simulink model "e11_cascade"  (R2020a)
settings: Solver=FixedStepAuto  StartTime=0.0  StopTime=options.T_train  RelTol=1e-3  AbsTol=1e-6
model workspace (MATLAB code in the model file):
  | scd_aero_guid_dat
undefined symbols (not defined in the file or in its folder): Cm_alpha, Cm_el, Cm_q, Cx_alpha, Cz_alpha, Cz_el, d_ref, DiscIntNeverNeededParam, g, h_ini, options, S_ref, Thrust, x_ini
libraries: neural x86, aerospace x6, simulink x1
(part 1 of 5)
settings Model: ExtModeTrigMode=oneshot  ExtModeArmWhenConnect=off  ExtModeAutoUpdateStatusClock=off  Creator=The MathWorks, Inc.  LastModifiedBy=kekatos
settings SolverCC: AutoScaleAbsTol=off
settings DataIOCC: SaveFormat=Array  SaveOutput=off  SignalLogging=off  SaveTime=off  ReturnWorkspaceOutputs=off  SignalLoggingName=sigsOut
settings OptimizationCC: BlockReduction=off  BooleanDataType=off  DefaultParameterBehavior=Inlined  InlineInvariantSignals=on  BufferReuse=off  ExpressionDepthLimit=2147483647  InitFltsAndDblsToZero=on  LifeSpan=inf
settings DebuggingCC: SaveWithParameterizedLinksMsg=none  UnderspecifiedInitializationDetection=Classic  MergeDetectMultiDrivingBlocksExec=none  CheckExecutionContextPreStartOutputMsg=on  CheckExecutionContextRuntimeOutputMsg=on  SignalResolutionControl=TryResolveAllWithWarning  MultiTaskDSMMsg=warning  FcnCallInpInsideContextMsg=warning  StateNameClashWarn=warning  SFUnexpectedBacktrackingDiag=warning  SFNoUnconditionalDefaultTransitionDiag=warning  SFExecutionAtInitializationDiag=none  ArithmeticOperatorsInVariantConditions=warning
settings HardwareCC: ProdBitPerPointer=32  ProdBitPerSizeT=32  ProdBitPerPtrDiffT=32  ProdLargestAtomicFloat=None  ProdIntDivRoundTo=Undefined  ProdEndianess=Unspecified  ProdWordSize=32  ProdHWDeviceType=32-bit Generic  TargetUnknown=on
settings ModelReferenceCC: UpdateModelReferenceTargets=IfOutOfDate  PropagateSignalLabelsOutOfModel=off
settings SFSimCC: SimUseLocalCustomCode=off  CustomCodeUndefinedFunction=UseInterfaceOnly
settings RTWCC: RTWUseLocalCustomCode=off
settings CodeAppCC: StateflowObjectComments=on
settings GRTTargetCC: TargetFcnLib=ansi_tfl_tmw.mat  TargetLangStandard=C89/C90 (ANSI)  CombineOutputUpdateFcns=off  GRTInterface=on
settings ConfigComp: CovMetricSettings=dw  CovHtmlReporting=on  CovSaveCumulativeToWorkspaceVar=on  CovSaveSingleToWorkspaceVar=on  CovExternalEMLEnable=off

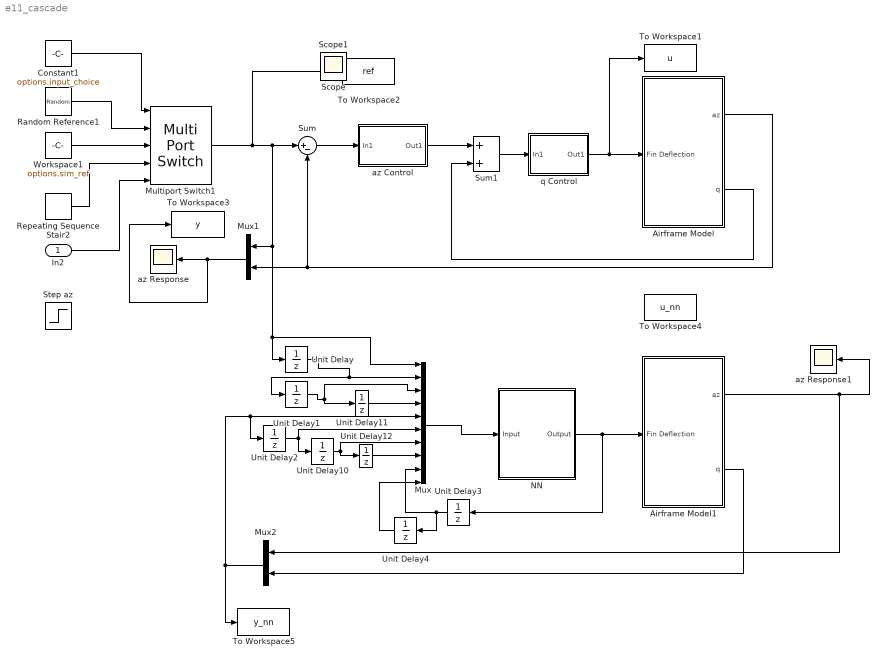
== system e11_cascade ==
  In2 : Inport
  Airframe Model : Subsystem
      settings: RTWMemSecFuncInitTerm=Default  RTWMemSecFuncExecute=Default  RTWMemSecDataConstants=Default  RTWMemSecDataInternal=Default  RTWMemSecDataParameters=Default
  Airframe Model1 : Subsystem
      settings: RTWMemSecFuncInitTerm=Default  RTWMemSecFuncExecute=Default  RTWMemSecDataConstants=Default  RTWMemSecDataInternal=Default  RTWMemSecDataParameters=Default
  Constant1 : Constant  Value=options.input_choice
  Multiport Switch1 : MultiPortSwitch  Inputs=4
  Mux : Mux  Inputs=10
  Mux1 : Mux  Inputs=2
  Mux2 : Mux  Inputs=2
  NN : Subsystem
      mask help: Feed-Forward Neural Network
      mask Display: e = 0.06;c1 = [120 150 230]/255;c2 = ([120 150 230]+0)/383;c3 = ([120 150 230]+128)/383;patch([0 1 1 0],[0 0 1 1],c1);patch([0 1 1 1-e 1-e 0+e],[0 0 1 1-e 0+e 0+e],c2);patch([0 0 1 1-e 0+e 0+e],[0 1 1 1-e 1-e 0+e],c3);plot([0 1 1 0 0],[0 0 1 1 0]);fprintf('NNET');port_label('input',1,' Input');port_label('output',1,'Output ');
  Random Reference1 : UniformRandomNumber  Minimum=options.ref_min  Maximum=options.ref_max  Seed=randi(2^32,[1 ])  SampleTime=options.ref_Ts
  Repeating Sequence Stair2 : simulink/Sources/Repeating Sequence Stair  OutValues=options.sim_cov  tsamp=options.ref_Ts  OutMin=[]  OutMax=[]  OutDataTypeStr=double  OutputDataTypeScalingMode=double  OutDataType=fixdt(0,8)  ConRadixGroup=Best Precision: Vector-wise  OutScaling=2^-12
  Step az : Step  After=200  SampleTime=0
  Sum : Sum  Inputs=|+-  SaturateOnIntegerOverflow=on
  Sum1 : Sum  SaturateOnIntegerOverflow=on
  To Workspace1 : ToWorkspace  VariableName=u  SaveFormat=Structure With Time  SampleTime=options.dt
  To Workspace2 : ToWorkspace  VariableName=ref  SaveFormat=Structure With Time  SampleTime=options.dt
  To Workspace3 : ToWorkspace  VariableName=y  SaveFormat=Structure With Time  SampleTime=options.dt
  To Workspace4 : ToWorkspace  VariableName=u_nn  SaveFormat=Structure With Time  SampleTime=options.dt
  To Workspace5 : ToWorkspace  VariableName=y_nn  SaveFormat=Structure With Time  SampleTime=options.dt
  Unit Delay{,1..4,10..12} (8 alike) : UnitDelay  SampleTime=-1  HasFrameUpgradeWarning=on
  Workspace1 : Constant  Value=options.sim_ref
  az Control : Subsystem
      settings: RTWMemSecFuncInitTerm=Default  RTWMemSecFuncExecute=Default  RTWMemSecDataConstants=Default  RTWMemSecDataInternal=Default  RTWMemSecDataParameters=Default
  az Response : Scope
  az Response1 : Scope
  q Control : Subsystem
      settings: RTWMemSecFuncInitTerm=Default  RTWMemSecFuncExecute=Default  RTWMemSecDataConstants=Default  RTWMemSecDataInternal=Default  RTWMemSecDataParameters=Default
  Scope : Scope
  Scope1 : Scope
  wires:
  Airframe Model/2(q) -> Sum1/2
  Sum1/1 -> q Control/1(In1)
  Airframe Model/1(az) -> Sum/2, Mux1/2
  Mux1/1 -> To Workspace3/1, az Response/1
  az Control/1(Out1) -> Sum1/1
  q Control/1(Out1) -> To Workspace1/1, Airframe Model/1(Fin Deflection)
  Sum/1 -> az Control/1(In1)
  Repeating Sequence Stair2/1 -> Multiport Switch1/4
  Random Reference1/1 -> Multiport Switch1/2
  In2/1 -> Multiport Switch1/5
  Workspace1/1 -> Multiport Switch1/3
  Constant1/1 -> Multiport Switch1/1
  Airframe Model1/2(q) -> Mux2/2
  Mux2/1 -> Unit Delay2/1, Mux/5, To Workspace5/1
  Unit Delay10/1 -> Mux/7, Unit Delay12/1
  Multiport Switch1/1 -> To Workspace2/1, Sum/1, Mux/1, Unit Delay/1, Mux1/1
  Unit Delay3/1 -> Mux/9, Unit Delay4/1
  Unit Delay1/1 -> Unit Delay11/1, Mux/3
  Unit Delay2/1 -> Mux/6, Unit Delay10/1
  Unit Delay/1 -> Unit Delay1/1, Mux/2
  NN/1(Output) -> Airframe Model1/1(Fin Deflection), Unit Delay3/1
  Mux/1 -> NN/1(Input)
  Unit Delay11/1 -> Mux/4
  Unit Delay12/1 -> Mux/8
  Unit Delay4/1 -> Mux/10
  Airframe Model1/1(az) -> az Response1/1, Mux2/1

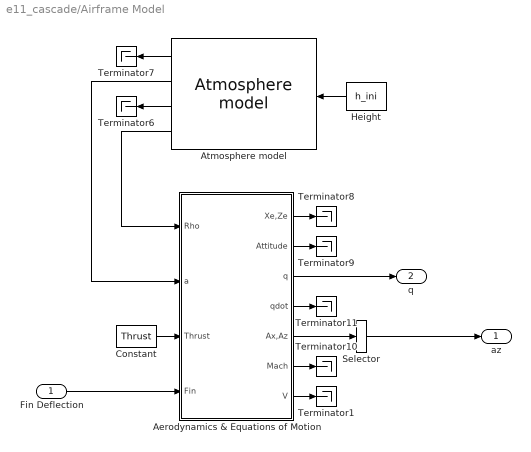
== system e11_cascade/Airframe Model ==
  Fin Deflection : Inport
  Aerodynamics & Equations of Motion : Subsystem
      settings: RTWMemSecFuncInitTerm=Default  RTWMemSecFuncExecute=Default  RTWMemSecDataConstants=Default  RTWMemSecDataInternal=Default  RTWMemSecDataParameters=Default
  Atmosphere model : aerospace/Atmosphere/Atmosphere model
      settings: SourceProductBaseCode=SL
  Constant : Constant  Value=Thrust
  Height : Constant  Value=h_ini
  Selector : Selector  InputPortWidth=2  IndexOptions=Index vector (dialog)  Indices=[2]  OutputSizes=1
  Terminator{1,6..11} (7 alike) : Terminator
  az : Outport  InitialOutput=0
  q : Outport  Port=2  InitialOutput=0
  wires:
  Height/1 -> Atmosphere model/1
  Atmosphere model/1 -> Terminator7/1
  Atmosphere model/3 -> Terminator6/1
  Constant/1 -> Aerodynamics & Equations of Motion/3(Thrust)
  Fin Deflection/1 -> Aerodynamics & Equations of Motion/4(Fin)
  Aerodynamics & Equations of Motion/1(Xe,Ze) -> Terminator8/1
  Aerodynamics & Equations of Motion/2(Attitude) -> Terminator9/1
  Aerodynamics & Equations of Motion/3(q) -> q/1
  Aerodynamics & Equations of Motion/4(qdot) -> Terminator11/1
  Aerodynamics & Equations of Motion/5(Ax,Az) -> Selector/1
  Aerodynamics & Equations of Motion/6(Mach) -> Terminator10/1
  Atmosphere model/4 -> Aerodynamics & Equations of Motion/1(Rho)
  Atmosphere model/2 -> Aerodynamics & Equations of Motion/2(a)
  Selector/1 -> az/1
  Aerodynamics & Equations of Motion/7(V) -> Terminator1/1

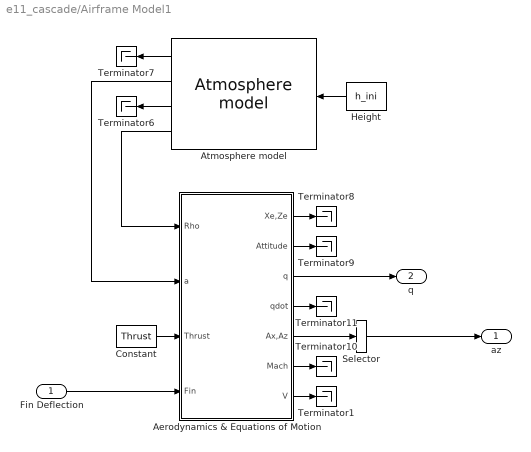
== system e11_cascade/Airframe Model1 ==
  Fin Deflection : Inport
  Aerodynamics & Equations of Motion : Subsystem
      settings: RTWMemSecFuncInitTerm=Default  RTWMemSecFuncExecute=Default  RTWMemSecDataConstants=Default  RTWMemSecDataInternal=Default  RTWMemSecDataParameters=Default
  Atmosphere model : aerospace/Atmosphere/Atmosphere model
      settings: SourceProductBaseCode=SL
  Constant : Constant  Value=Thrust
  Height : Constant  Value=h_ini
  Selector : Selector  InputPortWidth=2  IndexOptions=Index vector (dialog)  Indices=[2]  OutputSizes=1
  Terminator{1,6..11} (7 alike) : Terminator
  az : Outport  InitialOutput=0
  q : Outport  Port=2  InitialOutput=0
  wires:
  Aerodynamics & Equations of Motion/7(V) -> Terminator1/1
  Selector/1 -> az/1
  Atmosphere model/2 -> Aerodynamics & Equations of Motion/2(a)
  Atmosphere model/4 -> Aerodynamics & Equations of Motion/1(Rho)
  Aerodynamics & Equations of Motion/6(Mach) -> Terminator10/1
  Aerodynamics & Equations of Motion/5(Ax,Az) -> Selector/1
  Aerodynamics & Equations of Motion/4(qdot) -> Terminator11/1
  Aerodynamics & Equations of Motion/3(q) -> q/1
  Aerodynamics & Equations of Motion/2(Attitude) -> Terminator9/1
  Aerodynamics & Equations of Motion/1(Xe,Ze) -> Terminator8/1
  Fin Deflection/1 -> Aerodynamics & Equations of Motion/4(Fin)
  Constant/1 -> Aerodynamics & Equations of Motion/3(Thrust)
  Atmosphere model/3 -> Terminator6/1
  Atmosphere model/1 -> Terminator7/1
  Height/1 -> Atmosphere model/1

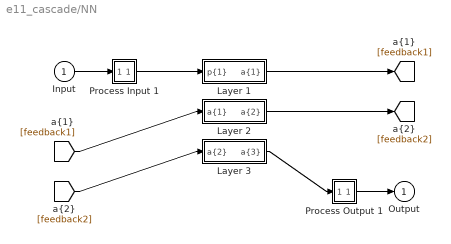
== system e11_cascade/NN ==
  Input : Inport  PortDimensions=14
      mask Display: e = 0.06;c1 = [120 230 180]/255;c2 = ([120 230 180]+0)/(256+128);c3 = ([120 230 180]+128)/(256+128);patch([0 1 1 0],[0 0 1 1],c1);patch([0 1 1 1-e 1-e 0+e],[0 0 1 1-e 0+e 0+e],c2);patch([0 0 1 1-e 0+e 0+e],[0 1 1 1-e 1-e 0+e],c3);plot([0 1 1 0 0],[0 0 1 1 0]);
  Layer 1 : Subsystem
      mask Display: e = 0.06;c1 = [120 150 230]/255;c2 = ([120 150 230]+0)/383;c3 = ([120 150 230]+128)/383;patch([0 1 1 0],[0 0 1 1],c1);patch([0 1 1 1-e 1-e 0+e],[0 0 1 1-e 0+e 0+e],c2);patch([0 0 1 1-e 0+e 0+e],[0 1 1 1-e 1-e 0+e],c3);plot([0 1 1 0 0],[0 0 1 1 0]);
  Layer 2 : Subsystem
      mask Display: e = 0.06;c1 = [120 150 230]/255;c2 = ([120 150 230]+0)/383;c3 = ([120 150 230]+128)/383;patch([0 1 1 0],[0 0 1 1],c1);patch([0 1 1 1-e 1-e 0+e],[0 0 1 1-e 0+e 0+e],c2);patch([0 0 1 1-e 0+e 0+e],[0 1 1 1-e 1-e 0+e],c3);plot([0 1 1 0 0],[0 0 1 1 0]);
  Layer 3 : Subsystem
      mask Display: e = 0.06;c1 = [120 150 230]/255;c2 = ([120 150 230]+0)/383;c3 = ([120 150 230]+128)/383;patch([0 1 1 0],[0 0 1 1],c1);patch([0 1 1 1-e 1-e 0+e],[0 0 1 1-e 0+e 0+e],c2);patch([0 0 1 1-e 0+e 0+e],[0 1 1 1-e 1-e 0+e],c3);plot([0 1 1 0 0],[0 0 1 1 0]);
  Process Input 1 : Subsystem
      mask Display: e = 0.06;c1 = [120 150 230]/255;c2 = ([120 150 230]+0)/383;c3 = ([120 150 230]+128)/383;patch([0 1 1 0],[0 0 1 1],c1);patch([0 1 1 1-e 1-e 0+e],[0 0 1 1-e 0+e 0+e],c2);patch([0 0 1 1-e 0+e 0+e],[0 1 1 1-e 1-e 0+e],c3);plot([0 1 1 0 0],[0 0 1 1 0]);
  Process Output 1 : Subsystem
      mask Display: e = 0.06;c1 = [120 150 230]/255;c2 = ([120 150 230]+0)/383;c3 = ([120 150 230]+128)/383;patch([0 1 1 0],[0 0 1 1],c1);patch([0 1 1 1-e 1-e 0+e],[0 0 1 1-e 0+e 0+e],c2);patch([0 0 1 1-e 0+e 0+e],[0 1 1 1-e 1-e 0+e],c3);plot([0 1 1 0 0],[0 0 1 1 0]);
  Output : Outport  InitialOutput=0
      mask Display: e = 0.06;c1 = [120 230 180]/255;c2 = ([120 230 180]+0)/(256+128);c3 = ([120 230 180]+128)/(256+128);patch([0 1 1 0],[0 0 1 1],c1);patch([0 1 1 1-e 1-e 0+e],[0 0 1 1-e 0+e 0+e],c2);patch([0 0 1 1-e 0+e 0+e],[0 1 1 1-e 1-e 0+e],c3);plot([0 1 1 0 0],[0 0 1 1 0]);
  wires:
  Input/1 -> Process Input 1/1(x)
  Process Output 1/1(y) -> Output/1
  Process Input 1/1(p) -> Layer 1/1("p{1}")
  Layer 1/1("a{1}") -> [feedback1]
  [feedback1] -> Layer 2/1("a{1} ")
  Layer 2/1("a{2}") -> [feedback2]
  [feedback2] -> Layer 3/1("a{2} ")
  Layer 3/1("a{3}") -> Process Output 1/1(a)

== system e11_cascade/az Control ==
  In1 : Inport
  Discrete-Time Integrator1 : DiscreteIntegrator  SampleTime=0.01  ICPrevOutput=DiscIntNeverNeededParam  ICPrevScaledInput=DiscIntNeverNeededParam
  az DTF : DiscreteTransferFcn  Numerator=[100.109745 -99.109745]  Denominator=[1 -0.88893]  SampleTime=0.01
  az Gain : Gain  Gain=0.00027507
  Out1 : Outport
  wires:
  az DTF/1 -> Discrete-Time Integrator1/1
  Discrete-Time Integrator1/1 -> az Gain/1
  In1/1 -> az DTF/1
  az Gain/1 -> Out1/1

== system e11_cascade/q Control ==
  In1 : Inport
  Discrete-Time Integrator : DiscreteIntegrator  SampleTime=0.01  ICPrevOutput=DiscIntNeverNeededParam  ICPrevScaledInput=DiscIntNeverNeededParam
  q Gain : Gain  Gain=2.7717622
  Out1 : Outport
  wires:
  Discrete-Time Integrator/1 -> q Gain/1
  In1/1 -> Discrete-Time Integrator/1
  q Gain/1 -> Out1/1

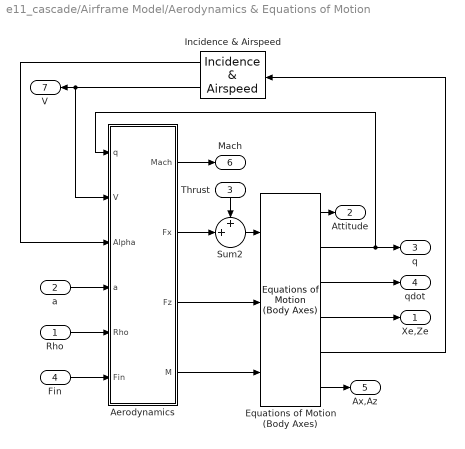
== system e11_cascade/Airframe Model/Aerodynamics & Equations of Motion ==
  Rho : Inport
  a : Inport  Port=2
  Thrust : Inport  Port=3
  Fin : Inport  Port=4
  " Equations of Motion (Body Axes)" : aerospace/3DoF Equations of Motion / Equations of Motion (Body Axes)  v_ini=v_ini  theta_ini=theta_ini  alpha_ini=alpha_ini  q_ini=q_ini  pos_ini=[x_ini -h_ini]  mass=mass  Iyy=Iyy  g=g
      settings: SourceProductBaseCode=SL
  Aerodynamics : Subsystem
      settings: RTWMemSecFuncInitTerm=Default  RTWMemSecFuncExecute=Default  RTWMemSecDataConstants=Default  RTWMemSecDataInternal=Default  RTWMemSecDataParameters=Default
  Incidence & Airspeed : aerospace/3DoF Equations of Motion /Incidence  & Airspeed
      settings: SourceProductBaseCode=SL
  Sum2 : Sum  Inputs=++|  InputSameDT=on  SaturateOnIntegerOverflow=on  OutDataTypeStr=Inherit: Same as first input
  Xe,Ze : Outport  InitialOutput=0
  Attitude : Outport  Port=2  InitialOutput=0
  q : Outport  Port=3  InitialOutput=0
  qdot : Outport  Port=4  InitialOutput=0
  Ax,Az : Outport  Port=5  InitialOutput=0
  Mach : Outport  Port=6  InitialOutput=0
  V : Outport  Port=7  InitialOutput=0
  wires:
  " Equations of Motion (Body Axes)"/5 -> Incidence & Airspeed/1
  " Equations of Motion (Body Axes)"/6 -> Ax,Az/1
  " Equations of Motion (Body Axes)"/4 -> Xe,Ze/1
  " Equations of Motion (Body Axes)"/1 -> Attitude/1
  " Equations of Motion (Body Axes)"/3 -> qdot/1
  " Equations of Motion (Body Axes)"/2 -> Aerodynamics/1(q), q/1
  Thrust/1 -> Sum2/1
  Aerodynamics/2(Fx) -> Sum2/2
  Aerodynamics/3(Fz) -> " Equations of Motion (Body Axes)"/2
  Incidence & Airspeed/2 -> Aerodynamics/2(V), V/1
  Fin/1 -> Aerodynamics/6(Fin)
  a/1 -> Aerodynamics/4(a)
  Rho/1 -> Aerodynamics/5(Rho)
  Incidence & Airspeed/1 -> Aerodynamics/3(Alpha)
  Sum2/1 -> " Equations of Motion (Body Axes)"/1
  Aerodynamics/4(" M") -> " Equations of Motion (Body Axes)"/3
  Aerodynamics/1(" Mach") -> Mach/1

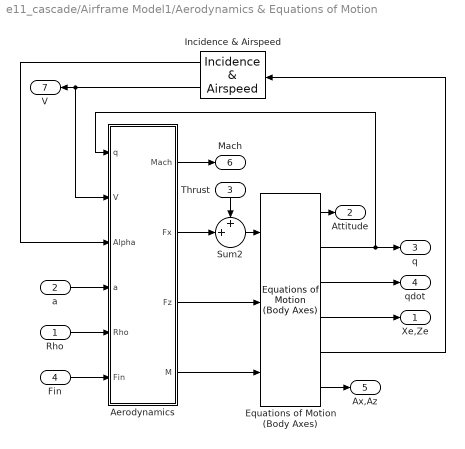
== system e11_cascade/Airframe Model1/Aerodynamics & Equations of Motion ==
  Rho : Inport
  a : Inport  Port=2
  Thrust : Inport  Port=3
  Fin : Inport  Port=4
  " Equations of Motion (Body Axes)" : aerospace/3DoF Equations of Motion / Equations of Motion (Body Axes)  v_ini=v_ini  theta_ini=theta_ini  alpha_ini=alpha_ini  q_ini=q_ini  pos_ini=[x_ini -h_ini]  mass=mass  Iyy=Iyy  g=g
      settings: SourceProductBaseCode=SL
  Aerodynamics : Subsystem
      settings: RTWMemSecFuncInitTerm=Default  RTWMemSecFuncExecute=Default  RTWMemSecDataConstants=Default  RTWMemSecDataInternal=Default  RTWMemSecDataParameters=Default
  Incidence & Airspeed : aerospace/3DoF Equations of Motion /Incidence  & Airspeed
      settings: SourceProductBaseCode=SL
  Sum2 : Sum  Inputs=++|  InputSameDT=on  SaturateOnIntegerOverflow=on  OutDataTypeStr=Inherit: Same as first input
  Xe,Ze : Outport  InitialOutput=0
  Attitude : Outport  Port=2  InitialOutput=0
  q : Outport  Port=3  InitialOutput=0
  qdot : Outport  Port=4  InitialOutput=0
  Ax,Az : Outport  Port=5  InitialOutput=0
  Mach : Outport  Port=6  InitialOutput=0
  V : Outport  Port=7  InitialOutput=0
  wires:
  Aerodynamics/1(" Mach") -> Mach/1
  Aerodynamics/4(" M") -> " Equations of Motion (Body Axes)"/3
  Sum2/1 -> " Equations of Motion (Body Axes)"/1
  Incidence & Airspeed/1 -> Aerodynamics/3(Alpha)
  Rho/1 -> Aerodynamics/5(Rho)
  a/1 -> Aerodynamics/4(a)
  Fin/1 -> Aerodynamics/6(Fin)
  Incidence & Airspeed/2 -> V/1, Aerodynamics/2(V)
  Aerodynamics/3(Fz) -> " Equations of Motion (Body Axes)"/2
  Aerodynamics/2(Fx) -> Sum2/2
  Thrust/1 -> Sum2/1
  " Equations of Motion (Body Axes)"/2 -> q/1, Aerodynamics/1(q)
  " Equations of Motion (Body Axes)"/3 -> qdot/1
  " Equations of Motion (Body Axes)"/1 -> Attitude/1
  " Equations of Motion (Body Axes)"/4 -> Xe,Ze/1
  " Equations of Motion (Body Axes)"/6 -> Ax,Az/1
  " Equations of Motion (Body Axes)"/5 -> Incidence & Airspeed/1

== system e11_cascade/NN/Layer 1 ==
  "p{1}" : Inport  PortDimensions=14
      mask Display: e = 0.06;c1 = [120 230 180]/255;c2 = ([120 230 180]+0)/(256+128);c3 = ([120 230 180]+128)/(256+128);patch([0 1 1 0],[0 0 1 1],c1);patch([0 1 1 1-e 1-e 0+e],[0 0 1 1-e 0+e 0+e],c2);patch([0 0 1 1-e 0+e 0+e],[0 1 1 1-e 1-e 0+e],c3);plot([0 1 1 0 0],[0 0 1 1 0]);
  Delays 1 : Subsystem
      mask Display: e = 0.06;c1 = [120 150 230]/255;c2 = ([120 150 230]+0)/383;c3 = ([120 150 230]+128)/383;patch([0 1 1 0],[0 0 1 1],c1);patch([0 1 1 1-e 1-e 0+e],[0 0 1 1-e 0+e 0+e],c2);patch([0 0 1 1-e 0+e 0+e],[0 1 1 1-e 1-e 0+e],c3);plot([0 1 1 0 0],[0 0 1 1 0]);disp('0');
  "IW{1,1}" : Subsystem
      mask Display: e = 0.06;c1 = [120 150 230]/255;c2 = ([120 150 230]+0)/383;c3 = ([120 150 230]+128)/383;patch([0 1 1 0],[0 0 1 1],c1);patch([0 1 1 1-e 1-e 0+e],[0 0 1 1-e 0+e 0+e],c2);patch([0 0 1 1-e 0+e 0+e],[0 1 1 1-e 1-e 0+e],c3);plot([0 1 1 0 0],[0 0 1 1 0]);disp('W');
  "b{1}" : Constant  Value=[-1.8821708534062049356094803442829288542270660400390625;-1.802460432566146408817076007835566997528076171875;-1.7530059677640483783989111543633043766021728515625;-1.6724305438301225734676336287520825862884521484375;1.5849498454034216532448908765218220651149749755859375;-1.5345923051837069284175640859757550060749053955078125;1.4943782984250912893031681960565038025379180908203125;1.4160905478492080700192445874563418328762054443359375;1.4196287910000358056805680462275631725788116455078125;-1.3007242237567362419525807126774452626705169677734375;1.22985859289517041048611645237542688846588134765625;-1.221991582134111187230018913396634161472320556640625;1.1238083924645867472946747511741705238819122314453125;1.0596020677591251324400900557520799338817596435546875;-0.9762754001642530710114442626945674419403076171875;0.91877406579176856826762787022744305431842803955078125;-0.85578331273051022609621441006311215460300445556640625;0.8147419133835269722254679436446167528629302978515625;0.70936116877356047982772224713698960840702056884765625;-0.6583130293505521368757626987644471228122711181640625;0.58331635159070660545665987228858284652233123779296875;-0.53844687123000667394734364279429428279399871826171875;-0.474864988205371985063862894094199873507022857666015625;0.3907096477484881535957583764684386551380157470703125;-0.3616173561991582463548411396914161741733551025390625;-0.2496474324121536747522753785233362577855587005615234375;-0.2197250125343665205779331017765798605978488922119140625;-0.1502530598150421392578124368810676969587802886962890625;-0.09926020248688670333248040833495906554162502288818359375;0.04074025860001449783620586231336346827447414398193359375;0.0238502725048951348674197703303434536792337894439697265625;-0.03789917961798151824215352689861902035772800445556640625;-0.1228527887855924982662969568991684354841709136962890625;0.2208877237806216309312645762474858202040195465087890625;0.26240193244785336990076984875486232340335845947265625;0.333369622158970868586180813508690334856510162353515625;0.4126499981154634344449050331604667007923126220703125;-0.5019524380934552443278562350315041840076446533203125;0.51692103701853342467842367113917134702205657958984375;0.53365526482920255801900566439144313335418701171875;0.688971494119760219376757959253154695034027099609375;-0.6783078511763760420905100545496679842472076416015625;-0.79797313628244381789045291952788829803466796875;0.8524580366653593532788590891868807375431060791015625;-0.9077337344884546244117018432007171213626861572265625;-1.0179137258568278223691550010698847472667694091796875;1.0984340025720993327951191531610675156116485595703125;-1.09071528675166096178372754366137087345123291015625;1.17861563692017323745631074416451156139373779296875;-1.26571113630274023620359002961777150630950927734375;1.3134797250146583724728088782285340130329132080078125;-1.3729675744611586907240052823908627033233642578125;-1.4889344023807893346855735217104665935039520263671875;1.49093438571294445438297771033830940723419189453125;-1.57422363610492421770459259278140962123870849609375;-1.63116516779454467922505500609986484050750732421875;-1.6869112319489720785981035078293643891811370849609375;1.754488235700125908778090888517908751964569091796875;1.8047181838588020053038007972645573318004608154296875;1.9007665506672968280810209762421436607837677001953125]
      mask Display: e = 0.06;c1 = [120 150 230]/255;c2 = ([120 150 230]+0)/383;c3 = ([120 150 230]+128)/383;patch([0 1 1 0],[0 0 1 1],c1);patch([0 1 1 1-e 1-e 0+e],[0 0 1 1-e 0+e 0+e],c2);patch([0 0 1 1-e 0+e 0+e],[0 1 1 1-e 1-e 0+e],c3);plot([0 1 1 0 0],[0 0 1 1 0]);disp('b');
  netsum : Sum  Inputs=2  InputSameDT=on  SaturateOnIntegerOverflow=on  OutDataTypeStr=Inherit: Same as first input
      mask Display: e = 0.06;c1 = [120 150 230]/255;c2 = ([120 150 230]+0)/383;c3 = ([120 150 230]+128)/383;patch([0 1 1 0],[0 0 1 1],c1);patch([0 1 1 1-e 1-e 0+e],[0 0 1 1-e 0+e 0+e],c2);patch([0 0 1 1-e 0+e 0+e],[0 1 1 1-e 1-e 0+e],c3);plot([0 1 1 0 0],[0 0 1 1 0]);disp('+');
  tansig : neural/Transfer Functions/tansig
  "a{1}" : Outport  InitialOutput=[0;0;0;0;0;0;0;0;0;0;0;0;0;0;0;0;0;0;0;0;0;0;0;0;0;0;0;0;0;0;0;0;0;0;0;0;0;0;0;0;0;0;0;0;0;0;0;0;0;0;0;0;0;0;0;0;0;0;0;0]
      mask Display: e = 0.06;c1 = [120 230 180]/255;c2 = ([120 230 180]+0)/(256+128);c3 = ([120 230 180]+128)/(256+128);patch([0 1 1 0],[0 0 1 1],c1);patch([0 1 1 1-e 1-e 0+e],[0 0 1 1-e 0+e 0+e],c2);patch([0 0 1 1-e 0+e 0+e],[0 1 1 1-e 1-e 0+e],c3);plot([0 1 1 0 0],[0 0 1 1 0]);
  wires:
  "p{1}"/1 -> Delays 1/1("p{1}")
  Delays 1/1("pd{1,1}") -> "IW{1,1}"/1("pd{1,1}")
  "IW{1,1}"/1("iz{1,1}") -> netsum/1
  "b{1}"/1 -> netsum/2
  netsum/1 -> tansig/1
  tansig/1 -> "a{1}"/1

== system e11_cascade/NN/Layer 2 ==
  "a{1} " : Inport  PortDimensions=60
      mask Display: e = 0.06;c1 = [120 230 180]/255;c2 = ([120 230 180]+0)/(256+128);c3 = ([120 230 180]+128)/(256+128);patch([0 1 1 0],[0 0 1 1],c1);patch([0 1 1 1-e 1-e 0+e],[0 0 1 1-e 0+e 0+e],c2);patch([0 0 1 1-e 0+e 0+e],[0 1 1 1-e 1-e 0+e],c3);plot([0 1 1 0 0],[0 0 1 1 0]);
  Delays 1 : Subsystem
      mask Display: e = 0.06;c1 = [120 150 230]/255;c2 = ([120 150 230]+0)/383;c3 = ([120 150 230]+128)/383;patch([0 1 1 0],[0 0 1 1],c1);patch([0 1 1 1-e 1-e 0+e],[0 0 1 1-e 0+e 0+e],c2);patch([0 0 1 1-e 0+e 0+e],[0 1 1 1-e 1-e 0+e],c3);plot([0 1 1 0 0],[0 0 1 1 0]);disp('0');
  "LW{2,1}" : Subsystem
      mask Display: e = 0.06;c1 = [120 150 230]/255;c2 = ([120 150 230]+0)/383;c3 = ([120 150 230]+128)/383;patch([0 1 1 0],[0 0 1 1],c1);patch([0 1 1 1-e 1-e 0+e],[0 0 1 1-e 0+e 0+e],c2);patch([0 0 1 1-e 0+e 0+e],[0 1 1 1-e 1-e 0+e],c3);plot([0 1 1 0 0],[0 0 1 1 0]);disp('W');
  "b{2}" : Constant  Value=[1.46726911679936478094532503746449947357177734375;-1.3080031929047553074241250214981846511363983154296875;1.1978954308241396287115776431164704263210296630859375;1.0171923417914274789808359855669550597667694091796875;-0.89569091758998353736132003177772276103496551513671875;-0.7184613780716111453017447274760343134403228759765625;0.5615705577772429624161532046855427324771881103515625;0.383927309489718260326895915568456985056400299072265625;0.2243473674345659862883195501126465387642383575439453125;0.080110299885182867374311399544239975512027740478515625;-0.08247198323127913344166017850511707365512847900390625;0.2126748596837468030518181194565840996801853179931640625;-0.3714977852351031284428017897880636155605316162109375;-0.5347978741931618262839265298680402338504791259765625;0.71190677164888838124312542277039028704166412353515625;-0.85685460255502732263011012037168256938457489013671875;0.99467863264792522048907130738371051847934722900390625;-1.161879696304514819615860687918029725551605224609375;-1.3258550413531609013517709172447212040424346923828125;1.497804336936940927671457757242023944854736328125]
      mask Display: e = 0.06;c1 = [120 150 230]/255;c2 = ([120 150 230]+0)/383;c3 = ([120 150 230]+128)/383;patch([0 1 1 0],[0 0 1 1],c1);patch([0 1 1 1-e 1-e 0+e],[0 0 1 1-e 0+e 0+e],c2);patch([0 0 1 1-e 0+e 0+e],[0 1 1 1-e 1-e 0+e],c3);plot([0 1 1 0 0],[0 0 1 1 0]);disp('b');
  netsum : Sum  Inputs=2  InputSameDT=on  SaturateOnIntegerOverflow=on  OutDataTypeStr=Inherit: Same as first input
      mask Display: e = 0.06;c1 = [120 150 230]/255;c2 = ([120 150 230]+0)/383;c3 = ([120 150 230]+128)/383;patch([0 1 1 0],[0 0 1 1],c1);patch([0 1 1 1-e 1-e 0+e],[0 0 1 1-e 0+e 0+e],c2);patch([0 0 1 1-e 0+e 0+e],[0 1 1 1-e 1-e 0+e],c3);plot([0 1 1 0 0],[0 0 1 1 0]);disp('+');
  tansig : neural/Transfer Functions/tansig
  "a{2}" : Outport  InitialOutput=[0;0;0;0;0;0;0;0;0;0;0;0;0;0;0;0;0;0;0;0]
      mask Display: e = 0.06;c1 = [120 230 180]/255;c2 = ([120 230 180]+0)/(256+128);c3 = ([120 230 180]+128)/(256+128);patch([0 1 1 0],[0 0 1 1],c1);patch([0 1 1 1-e 1-e 0+e],[0 0 1 1-e 0+e 0+e],c2);patch([0 0 1 1-e 0+e 0+e],[0 1 1 1-e 1-e 0+e],c3);plot([0 1 1 0 0],[0 0 1 1 0]);
  wires:
  "a{1} "/1 -> Delays 1/1("p{2}")
  Delays 1/1("pd{2,1}") -> "LW{2,1}"/1("ad{2,1}")
  "LW{2,1}"/1("lz{2,1}") -> netsum/1
  "b{2}"/1 -> netsum/2
  netsum/1 -> tansig/1
  tansig/1 -> "a{2}"/1

== system e11_cascade/NN/Layer 3 ==
  "a{2} " : Inport  PortDimensions=20
      mask Display: e = 0.06;c1 = [120 230 180]/255;c2 = ([120 230 180]+0)/(256+128);c3 = ([120 230 180]+128)/(256+128);patch([0 1 1 0],[0 0 1 1],c1);patch([0 1 1 1-e 1-e 0+e],[0 0 1 1-e 0+e 0+e],c2);patch([0 0 1 1-e 0+e 0+e],[0 1 1 1-e 1-e 0+e],c3);plot([0 1 1 0 0],[0 0 1 1 0]);
  Delays 1 : Subsystem
      mask Display: e = 0.06;c1 = [120 150 230]/255;c2 = ([120 150 230]+0)/383;c3 = ([120 150 230]+128)/383;patch([0 1 1 0],[0 0 1 1],c1);patch([0 1 1 1-e 1-e 0+e],[0 0 1 1-e 0+e 0+e],c2);patch([0 0 1 1-e 0+e 0+e],[0 1 1 1-e 1-e 0+e],c3);plot([0 1 1 0 0],[0 0 1 1 0]);disp('0');
  "LW{3,2}" : Subsystem
      mask Display: e = 0.06;c1 = [120 150 230]/255;c2 = ([120 150 230]+0)/383;c3 = ([120 150 230]+128)/383;patch([0 1 1 0],[0 0 1 1],c1);patch([0 1 1 1-e 1-e 0+e],[0 0 1 1-e 0+e 0+e],c2);patch([0 0 1 1-e 0+e 0+e],[0 1 1 1-e 1-e 0+e],c3);plot([0 1 1 0 0],[0 0 1 1 0]);disp('W');
  "b{3}" : Constant  Value=-0.639518639566905466864454865572042763233184814453125
      mask Display: e = 0.06;c1 = [120 150 230]/255;c2 = ([120 150 230]+0)/383;c3 = ([120 150 230]+128)/383;patch([0 1 1 0],[0 0 1 1],c1);patch([0 1 1 1-e 1-e 0+e],[0 0 1 1-e 0+e 0+e],c2);patch([0 0 1 1-e 0+e 0+e],[0 1 1 1-e 1-e 0+e],c3);plot([0 1 1 0 0],[0 0 1 1 0]);disp('b');
  netsum : Sum  Inputs=2  InputSameDT=on  SaturateOnIntegerOverflow=on  OutDataTypeStr=Inherit: Same as first input
      mask Display: e = 0.06;c1 = [120 150 230]/255;c2 = ([120 150 230]+0)/383;c3 = ([120 150 230]+128)/383;patch([0 1 1 0],[0 0 1 1],c1);patch([0 1 1 1-e 1-e 0+e],[0 0 1 1-e 0+e 0+e],c2);patch([0 0 1 1-e 0+e 0+e],[0 1 1 1-e 1-e 0+e],c3);plot([0 1 1 0 0],[0 0 1 1 0]);disp('+');
  purelin : neural/Transfer Functions/purelin
  "a{3}" : Outport  InitialOutput=0
      mask Display: e = 0.06;c1 = [120 230 180]/255;c2 = ([120 230 180]+0)/(256+128);c3 = ([120 230 180]+128)/(256+128);patch([0 1 1 0],[0 0 1 1],c1);patch([0 1 1 1-e 1-e 0+e],[0 0 1 1-e 0+e 0+e],c2);patch([0 0 1 1-e 0+e 0+e],[0 1 1 1-e 1-e 0+e],c3);plot([0 1 1 0 0],[0 0 1 1 0]);
  wires:
  "a{2} "/1 -> Delays 1/1("p{3}")
  Delays 1/1("pd{3,2}") -> "LW{3,2}"/1("ad{3,2}")
  "LW{3,2}"/1("lz{3,2}") -> netsum/1
  "b{3}"/1 -> netsum/2
  netsum/1 -> purelin/1
  purelin/1 -> "a{3}"/1

== system e11_cascade/NN/Process Input 1 ==
  x : Inport  PortDimensions=14
      mask Display: e = 0.06;c1 = [120 230 180]/255;c2 = ([120 230 180]+0)/(256+128);c3 = ([120 230 180]+128)/(256+128);patch([0 1 1 0],[0 0 1 1],c1);patch([0 1 1 1-e 1-e 0+e],[0 0 1 1-e 0+e 0+e],c2);patch([0 0 1 1-e 0+e 0+e],[0 1 1 1-e 1-e 0+e],c3);plot([0 1 1 0 0],[0 0 1 1 0]);
  mapminmax : neural/Processing Functions/mapminmax  xmin=[150.811257688657860853709280491;0;0;0;150.811257688657860853709280491;-4.40198849792837698657876899233;0;-4.40198849792837698657876899233;0;-4.40198849792837698657876899233;0;-4.40198849792837698657876899233;0;0]  xmax=[199.797483783560863912498462014;199.797483783560863912498462014;199.797483783560863912498462014;199.797483783560863912498462014;199.797483783560863912498462014;200.008755309697249913369887508;199.797483783560863912498462014;200.008755309697249913369887508;199.797483783560863912498462014;200.008755309697249913369887508;199.797483783560863912498462014;200.008755309697249913369887508;0.20547017129288558390243224494;0.203980769093067837438582046161]  ymin=-1  ymax=1
  p : Outport  PortDimensions=14
      mask Display: e = 0.06;c1 = [120 230 180]/255;c2 = ([120 230 180]+0)/(256+128);c3 = ([120 230 180]+128)/(256+128);patch([0 1 1 0],[0 0 1 1],c1);patch([0 1 1 1-e 1-e 0+e],[0 0 1 1-e 0+e 0+e],c2);patch([0 0 1 1-e 0+e 0+e],[0 1 1 1-e 1-e 0+e],c3);plot([0 1 1 0 0],[0 0 1 1 0]);
  wires:
  x/1 -> mapminmax/1
  mapminmax/1 -> p/1

== system e11_cascade/NN/Process Output 1 ==
  a : Inport  PortDimensions=1
      mask Display: e = 0.06;c1 = [120 230 180]/255;c2 = ([120 230 180]+0)/(256+128);c3 = ([120 230 180]+128)/(256+128);patch([0 1 1 0],[0 0 1 1],c1);patch([0 1 1 1-e 1-e 0+e],[0 0 1 1-e 0+e 0+e],c2);patch([0 0 1 1-e 0+e 0+e],[0 1 1 1-e 1-e 0+e],c3);plot([0 1 1 0 0],[0 0 1 1 0]);
  mapminmax_reverse : neural/Processing Functions/mapminmax_reverse  xmin=0  xmax=0.206981800433038459763324112828  ymin=-1  ymax=1
  y : Outport  PortDimensions=1
      mask Display: e = 0.06;c1 = [120 230 180]/255;c2 = ([120 230 180]+0)/(256+128);c3 = ([120 230 180]+128)/(256+128);patch([0 1 1 0],[0 0 1 1],c1);patch([0 1 1 1-e 1-e 0+e],[0 0 1 1-e 0+e 0+e],c2);patch([0 0 1 1-e 0+e 0+e],[0 1 1 1-e 1-e 0+e],c3);plot([0 1 1 0 0],[0 0 1 1 0]);
  wires:
  a/1 -> mapminmax_reverse/1
  mapminmax_reverse/1 -> y/1

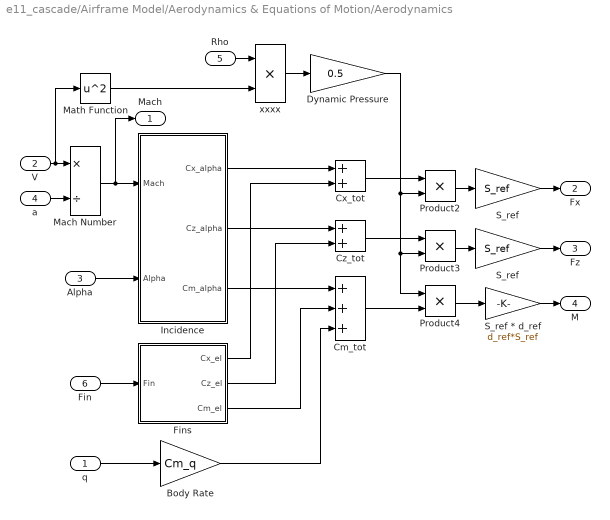
== system e11_cascade/Airframe Model/Aerodynamics & Equations of Motion/Aerodynamics ==
  q : Inport
  V : Inport  Port=2
  Alpha : Inport  Port=3
  a : Inport  Port=4
  Rho : Inport  Port=5
  Fin : Inport  Port=6
  Body Rate : Gain  Gain=Cm_q  SaturateOnIntegerOverflow=on  OutDataTypeStr=Inherit: Same as input  ParamDataTypeStr=Inherit: Same as input
  Cm_tot : Sum  Inputs=+++  InputSameDT=on  SaturateOnIntegerOverflow=on  OutDataTypeStr=Inherit: Same as first input
  Cx_tot : Sum  InputSameDT=on  SaturateOnIntegerOverflow=on  OutDataTypeStr=Inherit: Same as first input
  Cz_tot : Sum  InputSameDT=on  SaturateOnIntegerOverflow=on  OutDataTypeStr=Inherit: Same as first input
  Dynamic Pressure : Gain  Gain=0.5  SaturateOnIntegerOverflow=on  OutDataTypeStr=Inherit: Same as input  ParamDataTypeStr=Inherit: Same as input
  Fins : Subsystem
      settings: RTWMemSecFuncInitTerm=Default  RTWMemSecFuncExecute=Default  RTWMemSecDataConstants=Default  RTWMemSecDataInternal=Default  RTWMemSecDataParameters=Default
  Incidence : Subsystem
      settings: RTWMemSecFuncInitTerm=Default  RTWMemSecFuncExecute=Default  RTWMemSecDataConstants=Default  RTWMemSecDataInternal=Default  RTWMemSecDataParameters=Default
  Mach Number : Product  Inputs=*/  InputSameDT=on  SaturateOnIntegerOverflow=on  OutDataTypeStr=Inherit: Same as first input
  Math Function : Math  Operator=square  SignedPower=on  SaturateOnIntegerOverflow=on
  Product2 : Product  InputSameDT=on  SaturateOnIntegerOverflow=on  OutDataTypeStr=Inherit: Same as first input
  Product3 : Product  InputSameDT=on  SaturateOnIntegerOverflow=on  OutDataTypeStr=Inherit: Same as first input
  Product4 : Product  InputSameDT=on  SaturateOnIntegerOverflow=on  OutDataTypeStr=Inherit: Same as first input
  S_ref : Gain  Gain=S_ref  SaturateOnIntegerOverflow=on  OutDataTypeStr=Inherit: Same as input  ParamDataTypeStr=Inherit: Same as input
  S_ref * d_ref : Gain  Gain=d_ref*S_ref  SaturateOnIntegerOverflow=on  OutDataTypeStr=Inherit: Same as input  ParamDataTypeStr=Inherit: Same as input
  "S_ref " : Gain  Gain=S_ref  SaturateOnIntegerOverflow=on  OutDataTypeStr=Inherit: Same as input  ParamDataTypeStr=Inherit: Same as input
  xxxx : Product  InputSameDT=on  SaturateOnIntegerOverflow=on  OutDataTypeStr=Inherit: Same as first input
  " Mach" : Outport  InitialOutput=0
  Fx : Outport  Port=2  InitialOutput=[0]
  Fz : Outport  Port=3  InitialOutput=0
  " M" : Outport  Port=4  InitialOutput=0
  wires:
  Mach Number/1 -> Incidence/1(Mach), " Mach"/1
  q/1 -> Body Rate/1
  Cm_tot/1 -> Product4/2
  Product4/1 -> S_ref * d_ref/1
  S_ref * d_ref/1 -> " M"/1
  Fin/1 -> Fins/1(Fin)
  "S_ref "/1 -> Fz/1
  Product3/1 -> "S_ref "/1
  S_ref/1 -> Fx/1
  Product2/1 -> S_ref/1
  Cz_tot/1 -> Product3/1
  Cx_tot/1 -> Product2/1
  Alpha/1 -> Incidence/2(Alpha)
  a/1 -> Mach Number/2
  Body Rate/1 -> Cm_tot/3
  Fins/3(Cm_el) -> Cm_tot/2
  Incidence/3(Cm_alpha) -> Cm_tot/1
  Fins/2(Cz_el) -> Cz_tot/2
  Incidence/2(Cz_alpha) -> Cz_tot/1
  Fins/1(Cx_el) -> Cx_tot/2
  Incidence/1(Cx_alpha) -> Cx_tot/1
  V/1 -> Mach Number/1, Math Function/1
  Dynamic Pressure/1 -> Product4/1, Product3/2, Product2/2
  xxxx/1 -> Dynamic Pressure/1
  Rho/1 -> xxxx/1
  Math Function/1 -> xxxx/2

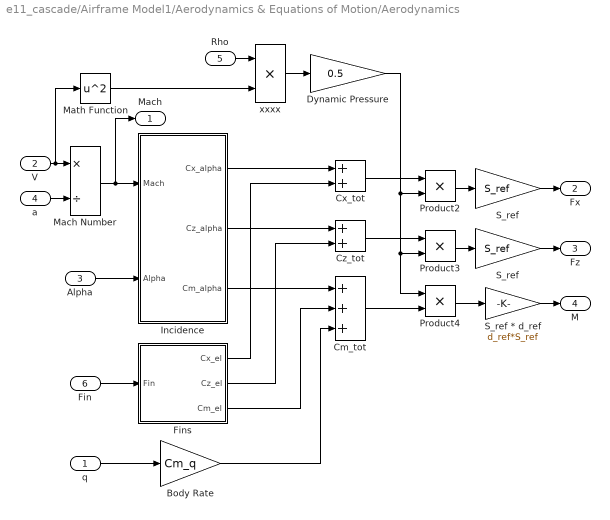
== system e11_cascade/Airframe Model1/Aerodynamics & Equations of Motion/Aerodynamics ==
  q : Inport
  V : Inport  Port=2
  Alpha : Inport  Port=3
  a : Inport  Port=4
  Rho : Inport  Port=5
  Fin : Inport  Port=6
  Body Rate : Gain  Gain=Cm_q  SaturateOnIntegerOverflow=on  OutDataTypeStr=Inherit: Same as input  ParamDataTypeStr=Inherit: Same as input
  Cm_tot : Sum  Inputs=+++  InputSameDT=on  SaturateOnIntegerOverflow=on  OutDataTypeStr=Inherit: Same as first input
  Cx_tot : Sum  InputSameDT=on  SaturateOnIntegerOverflow=on  OutDataTypeStr=Inherit: Same as first input
  Cz_tot : Sum  InputSameDT=on  SaturateOnIntegerOverflow=on  OutDataTypeStr=Inherit: Same as first input
  Dynamic Pressure : Gain  Gain=0.5  SaturateOnIntegerOverflow=on  OutDataTypeStr=Inherit: Same as input  ParamDataTypeStr=Inherit: Same as input
  Fins : Subsystem
      settings: RTWMemSecFuncInitTerm=Default  RTWMemSecFuncExecute=Default  RTWMemSecDataConstants=Default  RTWMemSecDataInternal=Default  RTWMemSecDataParameters=Default
  Incidence : Subsystem
      settings: RTWMemSecFuncInitTerm=Default  RTWMemSecFuncExecute=Default  RTWMemSecDataConstants=Default  RTWMemSecDataInternal=Default  RTWMemSecDataParameters=Default
  Mach Number : Product  Inputs=*/  InputSameDT=on  SaturateOnIntegerOverflow=on  OutDataTypeStr=Inherit: Same as first input
  Math Function : Math  Operator=square  SignedPower=on  SaturateOnIntegerOverflow=on
  Product2 : Product  InputSameDT=on  SaturateOnIntegerOverflow=on  OutDataTypeStr=Inherit: Same as first input
  Product3 : Product  InputSameDT=on  SaturateOnIntegerOverflow=on  OutDataTypeStr=Inherit: Same as first input
  Product4 : Product  InputSameDT=on  SaturateOnIntegerOverflow=on  OutDataTypeStr=Inherit: Same as first input
  S_ref : Gain  Gain=S_ref  SaturateOnIntegerOverflow=on  OutDataTypeStr=Inherit: Same as input  ParamDataTypeStr=Inherit: Same as input
  S_ref * d_ref : Gain  Gain=d_ref*S_ref  SaturateOnIntegerOverflow=on  OutDataTypeStr=Inherit: Same as input  ParamDataTypeStr=Inherit: Same as input
  "S_ref " : Gain  Gain=S_ref  SaturateOnIntegerOverflow=on  OutDataTypeStr=Inherit: Same as input  ParamDataTypeStr=Inherit: Same as input
  xxxx : Product  InputSameDT=on  SaturateOnIntegerOverflow=on  OutDataTypeStr=Inherit: Same as first input
  " Mach" : Outport  InitialOutput=0
  Fx : Outport  Port=2  InitialOutput=[0]
  Fz : Outport  Port=3  InitialOutput=0
  " M" : Outport  Port=4  InitialOutput=0
  wires:
  Math Function/1 -> xxxx/2
  Rho/1 -> xxxx/1
  xxxx/1 -> Dynamic Pressure/1
  Dynamic Pressure/1 -> Product2/2, Product3/2, Product4/1
  V/1 -> Math Function/1, Mach Number/1
  Incidence/1(Cx_alpha) -> Cx_tot/1
  Fins/1(Cx_el) -> Cx_tot/2
  Incidence/2(Cz_alpha) -> Cz_tot/1
  Fins/2(Cz_el) -> Cz_tot/2
  Incidence/3(Cm_alpha) -> Cm_tot/1
  Fins/3(Cm_el) -> Cm_tot/2
  Body Rate/1 -> Cm_tot/3
  a/1 -> Mach Number/2
  Alpha/1 -> Incidence/2(Alpha)
  Cx_tot/1 -> Product2/1
  Cz_tot/1 -> Product3/1
  Product2/1 -> S_ref/1
  S_ref/1 -> Fx/1
  Product3/1 -> "S_ref "/1
  "S_ref "/1 -> Fz/1
  Fin/1 -> Fins/1(Fin)
  S_ref * d_ref/1 -> " M"/1
  Product4/1 -> S_ref * d_ref/1
  Cm_tot/1 -> Product4/2
  q/1 -> Body Rate/1
  Mach Number/1 -> " Mach"/1, Incidence/1(Mach)

== system e11_cascade/NN/Layer 1/Delays 1 ==
  "p{1}" : Inport  PortDimensions=14
      mask Display: e = 0.06;c1 = [120 230 180]/255;c2 = ([120 230 180]+0)/(256+128);c3 = ([120 230 180]+128)/(256+128);patch([0 1 1 0],[0 0 1 1],c1);patch([0 1 1 1-e 1-e 0+e],[0 0 1 1-e 0+e 0+e],c2);patch([0 0 1 1-e 0+e 0+e],[0 1 1 1-e 1-e 0+e],c3);plot([0 1 1 0 0],[0 0 1 1 0]);
  mux : Mux  Inputs=1
      mask Display: e = 0.06;c1 = [120 150 230]/255;c2 = ([120 150 230]+0)/383;c3 = ([120 150 230]+128)/383;patch([0 1 1 0],[0 0 1 1],c1);patch([0 1 1 1-e 1-e 0+e],[0 0 1 1-e 0+e 0+e],c2);patch([0 0 1 1-e 0+e 0+e],[0 1 1 1-e 1-e 0+e],c3);plot([0 1 1 0 0],[0 0 1 1 0]);disp('Mux')
  "pd{1,1}" : Outport
      mask Display: e = 0.06;c1 = [120 230 180]/255;c2 = ([120 230 180]+0)/(256+128);c3 = ([120 230 180]+128)/(256+128);patch([0 1 1 0],[0 0 1 1],c1);patch([0 1 1 1-e 1-e 0+e],[0 0 1 1-e 0+e 0+e],c2);patch([0 0 1 1-e 0+e 0+e],[0 1 1 1-e 1-e 0+e],c3);plot([0 1 1 0 0],[0 0 1 1 0]);
  wires:
  "p{1}"/1 -> mux/1
  mux/1 -> "pd{1,1}"/1
